simulink model "Rotary_system_h_bridge_23a"  (R2023a)
settings: Solver=ode4  StartTime=0.0  StopTime=1  FixedStep=1e-6  RelTol=1e-3
InitFcn:
  | %% Parameters
  | 
  | param = struct();
  | 
  | % Volume of chambers
  | param.V1_0 = 1e-3;
  | param.V2_0 = 20e-6;
  | 
  | % Pressure rails
  | param.P_H = 20e6;
  | param.P_M = 10e6;
  | 
  | % Valve things
  | param.max_Avt = 0.5*0.25*pi*(20e-3)^2;
  | param.Cd = 0.6;
  | 
  | % Fluid properties
  | param.beta = 1.8e9;
  | param.rho = 870;
  | 
  | % Electric motor stuff
  | param.Kt = 70.5e-3;
  | param.Ke = 70.5e-3;
  | param.J_elec = 3000e-7;
  | 
  | % Pump things
  | param.J_hyd = 3000e-7;
  | param.hyd_D = 1.6e-6;    % In cc/rev
  | 
  | % Simulation time
  | T = 1.2;
settings Model: Creator=user  LastModifiedBy=ibrah408

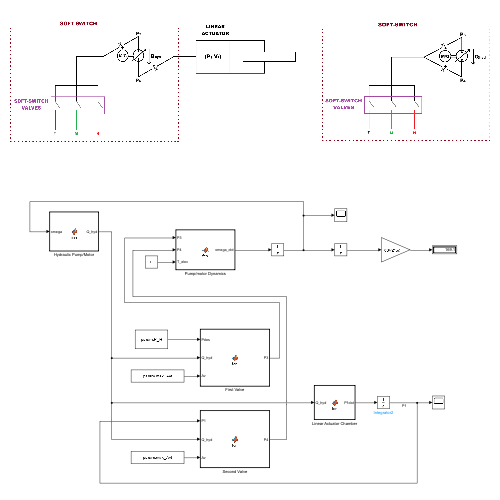
[thumbnail: Simulink's stored preview of the top-level diagram]
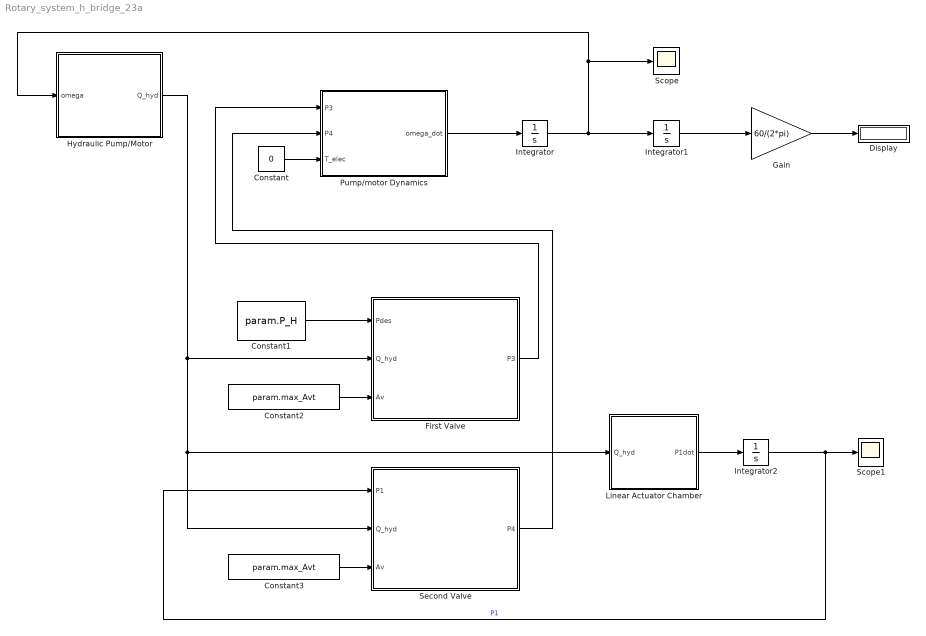
== system Rotary_system_h_bridge_23a ==
  Constant : Constant  Value=0
  Constant1 : Constant  Value=param.P_H
  Constant2 : Constant  Value=param.max_Avt
  Constant3 : Constant  Value=param.max_Avt
  Display : Display
  First Valve : MATLAB Function  TreatAsAtomicUnit=on
  Gain : Gain  Gain=60/(2*pi)
  Hydraulic Pump/Motor : MATLAB Function  TreatAsAtomicUnit=on
  Integrator : Integrator
  Integrator1 : Integrator
  Integrator2 : Integrator  InitialCondition=param.P_M
  Linear Actuator Chamber : MATLAB Function  TreatAsAtomicUnit=on
  Pump/motor Dynamics : MATLAB Function  TreatAsAtomicUnit=on
  Scope : Scope
  Scope1 : Scope
  Second Valve : MATLAB Function  TreatAsAtomicUnit=on
  wires:
  Constant/1 -> Pump/motor Dynamics/3(T_elec)
  Pump/motor Dynamics/1(omega_dot) -> Integrator/1
  Integrator/1 -> Integrator1/1, Hydraulic Pump/Motor/1(omega), Scope/1
  Integrator1/1 -> Gain/1
  Gain/1 -> Display/1
  Constant1/1 -> First Valve/1(Pdes)
  Hydraulic Pump/Motor/1(Q_hyd) -> Linear Actuator Chamber/1(Q_hyd), Second Valve/2(Q_hyd), First Valve/2(Q_hyd)
  Constant2/1 -> First Valve/3(Av)
  Constant3/1 -> Second Valve/3(Av)
  Linear Actuator Chamber/1(P1dot) -> Integrator2/1
  Integrator2/1 -> Second Valve/1(P1), Scope1/1  "P1"
  First Valve/1(P3) -> Pump/motor Dynamics/1(P3)
  Second Valve/1(P4) -> Pump/motor Dynamics/2(P4)

== matlab function Rotary_system_h_bridge_23a/Pump//motor Dynamics ==
  data: omega_dot output; P3 input; P4 input; param parameter; T_elec input
function omega_dot = fcn(P3, P4, param, T_elec)

hyd_torque = (param.hyd_D/(2*pi))*(P3-P4);
omega_dot = (1/(param.J_elec+param.J_hyd))*(hyd_torque - T_elec);

== matlab function Rotary_system_h_bridge_23a/Hydraulic Pump//Motor ==
  data: Q_hyd output; omega input; param parameter
function Q_hyd   = fcn(omega, param)

Q_hyd = (param.hyd_D/(2*pi))*omega;

== matlab function Rotary_system_h_bridge_23a/First Valve ==
  data: Pdes input; P3 output; Q_hyd input; Av input; param parameter
function P3 = fcn(Pdes, Q_hyd, Av, param)

K = param.Cd*Av*sqrt(2/param.rho);

P3 = Pdes - (Q_hyd/K)^2;

== matlab function Rotary_system_h_bridge_23a/Second Valve ==
  data: P1 input; P4 output; Q_hyd input; Av input; param parameter
function P4 = fcn(P1, Q_hyd, Av, param)

K = param.Cd*Av*sqrt(2/param.rho);
P4 = P1 + (Q_hyd/K)^2;

== matlab function Rotary_system_h_bridge_23a/Linear Actuator Chamber ==
  data: P1dot output; Q_hyd input; param parameter
function P1dot = fcn(Q_hyd, param)

P1dot = (param.beta/param.V1_0)*(Q_hyd);
